simulink model "Tirocinio4Parte1"  (R2025b)
settings: Solver=VariableStepAuto  StartTime=0.0  StopTime=150  RelTol=1e-6  AbsTol=1e-6
values from neighbouring files (symbols this model uses):
  M0 = 2    [Tirocinio4.m]
  M1 = [0 0 0 1/m1_2]'    [Tirocinio3.m]    (also in Tirocinio4.m = 0.5)
undefined symbols (not defined in the file or in its folder): A_comp, A_sys, B_comp, B_sys, C_comp, C_sys
libraries: simulink x1
settings Model: Creator=sarab  LastModifiedBy=Davide

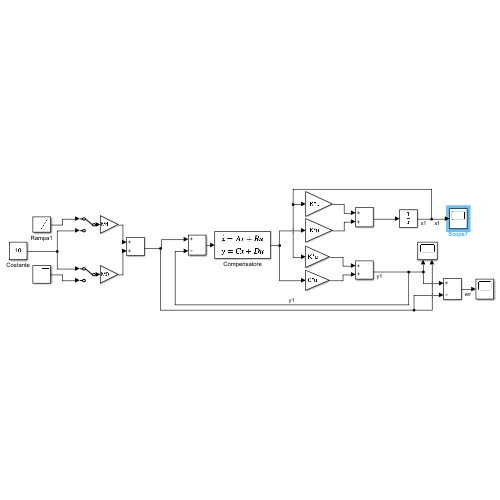
[thumbnail: Simulink's stored preview of the top-level diagram]
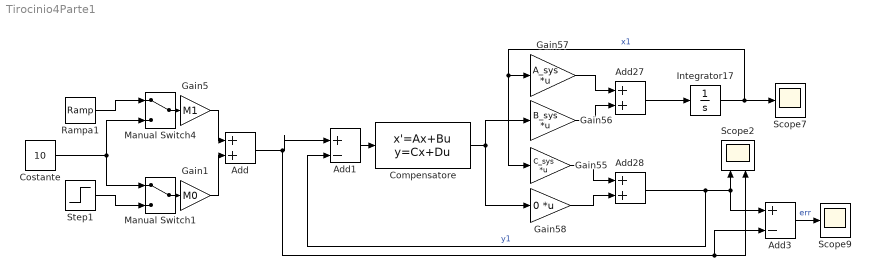
== system Tirocinio4Parte1 ==
  Add : Sum
  Add1 : Sum  Inputs=+|-
  Add27 : Sum
  Add28 : Sum
  Add3 : Sum  Inputs=+-
  Compensatore : StateSpace  A=A_comp  B=B_comp  C=C_comp  D=0  InitialCondition=0
  Costante : Constant  Value=10
  Gain1 : Gain  Gain=M0
  Gain5 : Gain  Gain=M1
  Gain55 : Gain  Gain=C_sys  Multiplication=Matrix(K*u)
  Gain56 : Gain  Gain=B_sys  Multiplication=Matrix(K*u)
  Gain57 : Gain  Gain=A_sys  Multiplication=Matrix(K*u)
  Gain58 : Gain  Gain=0  Multiplication=Matrix(K*u)
  Integrator17 : Integrator  InitialCondition=[0 0 0 0]  AbsoluteTolerance=1
  Manual Switch1 : ManualSwitch
  Manual Switch4 : ManualSwitch
  Rampa1 : simulink/Sources/Ramp  slope=1  start=0  InitialOutput=0
  Scope2 : Scope  NumInputPorts=2
      settings: ActiveDisplayYMinimum=-1.1432072829131599  ActiveDisplayYMaximum=38.539332399626517  DataLoggingVariableName=ScopeData5
  Scope7 : Scope
      settings: ActiveDisplayYMinimum=-5.4007810790739548  ActiveDisplayYMaximum=10.04120187056775  DataLoggingVariableName=ScopeData6
  Scope9 : Scope
      settings: ActiveDisplayYMinimum=-4.5710101672522338E-6  ActiveDisplayYMaximum=2.9213473504716876E-6  DataLoggingVariableName=ScopeData7
  Step1 : Step  Time=0  SampleTime=0
  wires:
  Rampa1/1 -> Manual Switch4/1
  Step1/1 -> Manual Switch1/2
  Costante/1 -> Manual Switch1/1, Manual Switch4/2
  Manual Switch1/1 -> Gain1/1
  Manual Switch4/1 -> Gain5/1
  Gain5/1 -> Add/1
  Gain1/1 -> Add/2
  Add/1 -> Scope2/2, Add3/2, Add1/1
  Add1/1 -> Compensatore/1
  Compensatore/1 -> Gain58/1, Gain56/1
  Gain57/1 -> Add27/1
  Gain56/1 -> Add27/2
  Add27/1 -> Integrator17/1
  Integrator17/1 -> Scope7/1, Gain55/1, Gain57/1  "x1"
  Gain55/1 -> Add28/1
  Gain58/1 -> Add28/2
  Add28/1 -> Add1/2, Scope2/1, Add3/1  "y1"
  Add3/1 -> Scope9/1  "err"
